simulink model "anim_tp_comde_NL"  (R2016a)
settings: Solver=ode5  SolverMode=SingleTasking  StartTime=0  StopTime=12  FixedStep=.005  MaxStep=0.02  RelTol=1e-3  AbsTol=1e-6
values from neighbouring files (symbols this model uses):
  F = acker(A,B,P)    [Model.m]
  K2 = -256/31.36    (= -8.16326530612)    [Model.m]
  L = 1    [Model.m]
  m = 0.5    [Model.m]
  M = 5    [Model.m]
undefined symbols (not defined in the file): g, X0
settings Model: Creator=user  LastModifiedBy=NADOUR
settings DataIOCC: ExternalInput=[]  InitialState=[]  SaveFormat=Array  SignalLoggingSaveFormat=ModelDataLogs  SaveOutput=off  SaveTime=off
settings OptimizationCC: BooleanDataType=off  ExpressionDepthLimit=2147483647  InitFltsAndDblsToZero=on
settings DebuggingCC: SaveWithParameterizedLinksMsg=none  UnderspecifiedInitializationDetection=Classic  MergeDetectMultiDrivingBlocksExec=none  SignalResolutionControl=TryResolveAllWithWarning  MultiTaskDSMMsg=warning  MultiTaskCondExecSysMsg=none  FcnCallInpInsideContextMsg=UseLocalSettings  StateNameClashWarn=warning
settings HardwareCC: ProdBitPerPointer=32  ProdLargestAtomicFloat=None  ProdIntDivRoundTo=Undefined  ProdEndianess=Unspecified  ProdWordSize=32  ProdHWDeviceType=32-bit Generic  TargetUnknown=on
settings ModelReferenceCC: PropagateSignalLabelsOutOfModel=off
settings GRTTargetCC: TargetFcnLib=ansi_tfl_tmw.mat  CombineOutputUpdateFcns=off  GRTInterface=on
settings ConfigComp: CovModelRefEnable=Off

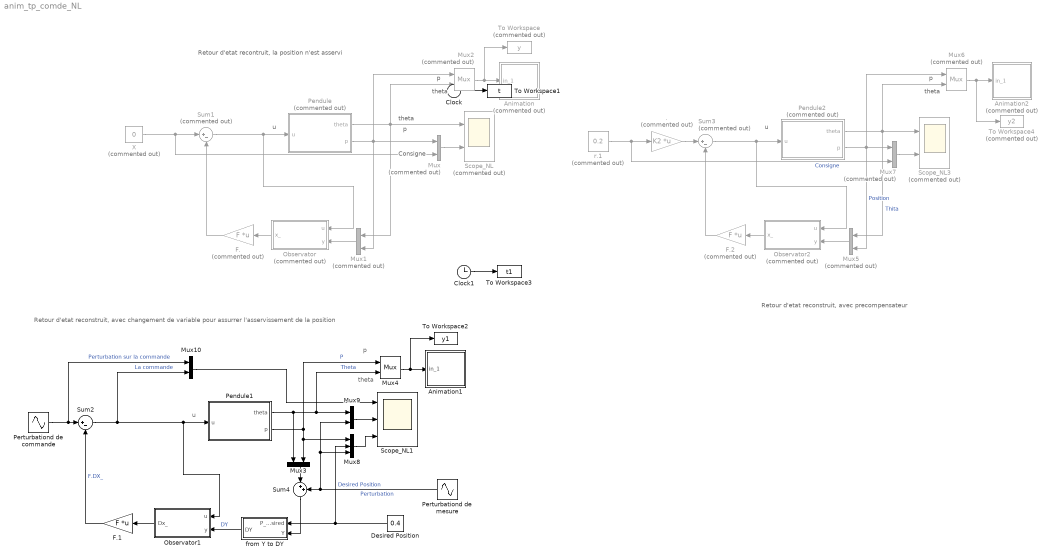
== system anim_tp_comde_NL ==
  note: Retour d'etat reconstruit, avec precompensateur
  note: Retour d'etat reconstruit, avec changement de variable pour assurrer l'asservissement de la position
  note: Retour d'etat recontruit, la position n'est asservi
  note: theta
  note: p
  note: theta
  note: p
  note: u
  note: Consigne
  note: theta
  note: p
  note: u
  note: theta
  note: p
  note: u
  . : Gain  Commented=on  Gain=K2  Multiplication=Matrix(K*u) (u vector)
  Animation : Subsystem  Commented=on  mask(Animation du déplacement du pendule inverse){}
      mask Help: Fonction d'animation du pendule inverse (voir s_fonction tp_pendan_g.m.
      mask Display: plot([-10 10],[0 0],[-2 -2 2 2],[0 1 1 0],[0 -3],[1 5])
  Animation1 : Subsystem  mask(Animation du déplacement du pendule inverse){}
      mask Help: Fonction d'animation du pendule inverse (voir s_fonction tp_pendan_g.m.
      mask Display: plot([-10 10],[0 0],[-2 -2 2 2],[0 1 1 0],[0 -3],[1 5])
  Animation2 : Subsystem  Commented=on  mask(Animation du déplacement du pendule inverse){}
      mask Help: Fonction d'animation du pendule inverse (voir s_fonction tp_pendan_g.m.
      mask Display: plot([-10 10],[0 0],[-2 -2 2 2],[0 1 1 0],[0 -3],[1 5])
  Clock : Clock
  Clock1 : Clock
  Desired Position : Constant  Value=0.4
  F. : Gain  Commented=on  Gain=F  Multiplication=Matrix(K*u) (u vector)
  F.1 : Gain  Gain=F  Multiplication=Matrix(K*u) (u vector)
  F.2 : Gain  Commented=on  Gain=F  Multiplication=Matrix(K*u) (u vector)
  Mux{,1..2,5..7} (6 alike) : Mux  Commented=on  Inputs=2
  Mux{3..4,9..10} (4 alike) : Mux  Inputs=2
  Mux8 : Mux  Inputs=3
  Observator : Subsystem  Commented=on
  Observator1 : Subsystem
  Observator2 : Subsystem  Commented=on
  Pendule : Subsystem  Commented=on  mask(Pendule inverse sur un chariot (éq. Non Linéaires)){M=M, m=m, l=L, g=g, x0=X0}
      mask prompts: M "Masse du chariot (kg):"; m "Masse du pendule (kg):"; l "Longueur de la barre (m):"; g "gravité (m/s^2):"; x0 "Conditions Initiales [theta theta' p p']"
      mask help: Utiliser le menu "Look under mask" pour voir les équations de la dynamique (celles de l'énoncé du TP)
      mask Help: Description Non Linéaire de la dynamique d'un pendule inverse sur un chariot.
      mask Display:
      | plot([-10 10],[1 1],[-2 -2 2 2],[1 2 2 1],[0 3],[2 5])
      | text(-13,0.5,'Eq. Non Linéaires')
      | plot([-14 14],[-0.5 -0.5])
  Pendule1 : Subsystem  mask(Pendule inverse sur un chariot (éq. Non Linéaires)){M=M, m=m, l=L, g=g, x0=X0}
      mask prompts: M "Masse du chariot (kg):"; m "Masse du pendule (kg):"; l "Longueur de la barre (m):"; g "gravité (m/s^2):"; x0 "Conditions Initiales [theta theta' p p']"
      mask help: Utiliser le menu "Look under mask" pour voir les équations de la dynamique (celles de l'énoncé du TP)
      mask Help: Description Non Linéaire de la dynamique d'un pendule inverse sur un chariot.
      mask Display:
      | plot([-10 10],[1 1],[-2 -2 2 2],[1 2 2 1],[0 3],[2 5])
      | text(-13,0.5,'Eq. Non Linéaires')
      | plot([-14 14],[-0.5 -0.5])
  Pendule2 : Subsystem  Commented=on  mask(Pendule inverse sur un chariot (éq. Non Linéaires)){M=M, m=m, l=L, g=g, x0=X0}
      mask prompts: M "Masse du chariot (kg):"; m "Masse du pendule (kg):"; l "Longueur de la barre (m):"; g "gravité (m/s^2):"; x0 "Conditions Initiales [theta theta' p p']"
      mask help: Utiliser le menu "Look under mask" pour voir les équations de la dynamique (celles de l'énoncé du TP)
      mask Help: Description Non Linéaire de la dynamique d'un pendule inverse sur un chariot.
      mask Display:
      | plot([-10 10],[1 1],[-2 -2 2 2],[1 2 2 1],[0 3],[2 5])
      | text(-13,0.5,'Eq. Non Linéaires')
      | plot([-14 14],[-0.5 -0.5])
  Perturbationd de commande : Sin  Amplitude=0.1  Frequency=0.1  SampleTime=0
  Perturbationd de mesure : Sin  Amplitude=0.2  Frequency=100  SampleTime=0
  Scope_NL : Scope  Commented=on  NumInputPorts=2
  Scope_NL1 : Scope  NumInputPorts=3
  Scope_NL3 : Scope  Commented=on  NumInputPorts=2
  Sum1 : Sum  Commented=on  Inputs=|+-
  Sum2 : Sum  Inputs=|+-
  Sum3 : Sum  Commented=on  Inputs=|+-
  Sum4 : Sum  Inputs=|++
  To Workspace : ToWorkspace  Commented=on  VariableName=y  SampleTime=0.1
  To Workspace1 : ToWorkspace  VariableName=t  SampleTime=0.1
  To Workspace2 : ToWorkspace  VariableName=y1  SampleTime=0.1
  To Workspace3 : ToWorkspace  VariableName=t1  SampleTime=0.1
  To Workspace4 : ToWorkspace  Commented=on  VariableName=y2  SampleTime=0.1
  X : Constant  Commented=on  Value=0
  from Y to DY : MATLAB Function  TreatAsAtomicUnit=on
  r.1 : Constant  Commented=on  Value=0.2
  wires:
  Mux2/1 -> To Workspace/1, Animation/1(in_1)
  Clock/1 -> To Workspace1/1
  Pendule/2(p) -> Mux/1, Mux1/2, Mux2/1
  Pendule/1(theta) -> Mux1/1, Mux2/2, Scope_NL/1
  Observator/1(x_) -> F./1
  Mux1/1 -> Observator/2(y)
  Sum1/1 -> Observator/1(u), Pendule/1(u)
  F./1 -> Sum1/2
  X/1 -> Mux/2, Sum1/1
  Mux4/1 -> To Workspace2/1, Animation1/1(in_1)
  Clock1/1 -> To Workspace3/1
  Pendule1/2(p) -> Mux8/1, Mux3/2, Mux4/1  "P"
  Pendule1/1(theta) -> Mux4/2, Mux9/1, Mux3/1  "Theta"
  Observator1/1(Dx_) -> F.1/1
  Sum4/1 -> from Y to DY/2(Y)
  Sum2/1 -> Mux10/2, Observator1/1(u), Pendule1/1(u)  "La commande"
  F.1/1 -> Sum2/2  "F.DX_"
  from Y to DY/1(DY) -> Observator1/2(y)  "DY"
  Desired Position/1 -> from Y to DY/1(P_desired), Mux8/2  "Desired Position"
  Mux6/1 -> Animation2/1(in_1), To Workspace4/1
  Pendule2/2(p) -> Mux5/2, Mux7/1, Mux6/1  "Position"
  Pendule2/1(theta) -> Mux5/1, Scope_NL3/1, Mux6/2  "Thita"
  Observator2/1(x_) -> F.2/1
  Mux5/1 -> Observator2/2(y)
  Sum3/1 -> Pendule2/1(u), Observator2/1(u)
  F.2/1 -> Sum3/2
  ./1 -> Sum3/1
  r.1/1 -> Mux7/2, ./1  "Consigne"
  Mux/1 -> Scope_NL/2
  Mux7/1 -> Scope_NL3/2
  Mux3/1 -> Sum4/1
  Perturbationd de mesure/1 -> Mux9/2, Mux8/3, Sum4/2  "Perturbation"
  Perturbationd de commande/1 -> Mux10/1, Sum2/1  "Perturbation sur la commande"
  Mux9/1 -> Scope_NL1/2
  Mux8/1 -> Scope_NL1/3
  Mux10/1 -> Scope_NL1/1

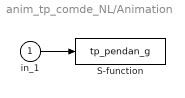
== system anim_tp_comde_NL/Animation ==
  in_1 : Inport
  S-function : S-Function  FunctionName=tp_pendan_g  SFunctionDeploymentMode=off  EnableBusSupport=off
      settings: DeleteFcn=pendan([],[],[],'DeleteBlock');
  wires:
  in_1/1 -> S-function/1

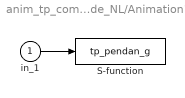
== system anim_tp_comde_NL/Animation1 ==
  in_1 : Inport
  S-function : S-Function  FunctionName=tp_pendan_g  SFunctionDeploymentMode=off  EnableBusSupport=off
      settings: DeleteFcn=pendan([],[],[],'DeleteBlock');
  wires:
  in_1/1 -> S-function/1

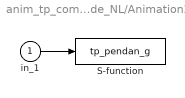
== system anim_tp_comde_NL/Animation2 ==
  in_1 : Inport
  S-function : S-Function  FunctionName=tp_pendan_g  SFunctionDeploymentMode=off  EnableBusSupport=off
      settings: DeleteFcn=pendan([],[],[],'DeleteBlock');
  wires:
  in_1/1 -> S-function/1

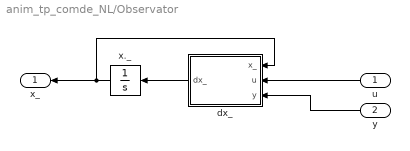
== system anim_tp_comde_NL/Observator ==
  u : Inport
  y : Inport  Port=2
  dx_ : MATLAB Function  TreatAsAtomicUnit=on
  x._ : Integrator
  x_ : Outport
  wires:
  u/1 -> dx_/2(u)
  y/1 -> dx_/3(y)
  dx_/1(dx_) -> x._/1
  x._/1 -> x_/1, dx_/1(x_)

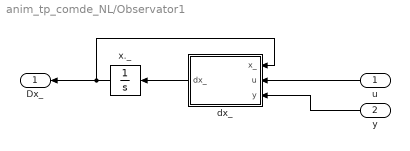
== system anim_tp_comde_NL/Observator1 ==
  u : Inport
  y : Inport  Port=2
  dx_ : MATLAB Function  TreatAsAtomicUnit=on
  x._ : Integrator
  Dx_ : Outport
  wires:
  u/1 -> dx_/2(u)
  y/1 -> dx_/3(y)
  dx_/1(dx_) -> x._/1
  x._/1 -> Dx_/1, dx_/1(x_)

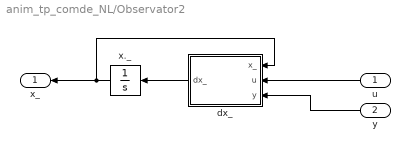
== system anim_tp_comde_NL/Observator2 ==
  u : Inport
  y : Inport  Port=2
  dx_ : MATLAB Function  TreatAsAtomicUnit=on
  x._ : Integrator
  x_ : Outport
  wires:
  x._/1 -> dx_/1(x_), x_/1
  dx_/1(dx_) -> x._/1
  y/1 -> dx_/3(y)
  u/1 -> dx_/2(u)

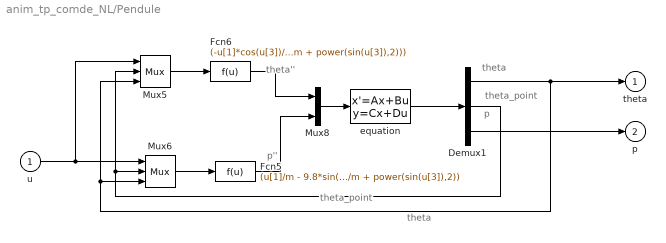
== system anim_tp_comde_NL/Pendule ==
  note: theta
  note: theta_point
  note: p''
  note: theta''
  note: theta
  note: theta_point
  note: p
  u : Inport
  Demux1 : Demux  Outputs=3
  Fcn5 : Fcn  Expr=(u[1]/m - 9.8*sin(u[3])*cos(u[3]) + L*power(u[2],2)*sin(u[3]))/(M/m + power(sin(u[3]),2))
  Fcn6 : Fcn  Expr=(-u[1]*cos(u[3])/m + (M+m)*9.8*sin(u[3])/m - L*power(u[2],2)*sin(u[3])*cos(u[3]))/(l*(M/m + power(sin(u[3]),2)))
  Mux5 : Mux  Inputs=3
  Mux6 : Mux  Inputs=3
  Mux8 : Mux  Inputs=2
  equation : StateSpace  A=[ 0 1 0 0 ; 0 0 0 0 ; 0 0 0 1; 0 0 0 0]  B=[0 0 ; 1 0 ; 0 0 ; 0 1]  C=[1 0 0 0 ; 0 1 0 0 ; 0 0 1 0]  D=zeros(3,2)  X0=x0
  theta : Outport  InitialOutput=0
  p : Outport  Port=2  InitialOutput=0
  wires:
  u/1 -> Mux6/1, Mux5/1
  Mux6/1 -> Fcn5/1
  Mux5/1 -> Fcn6/1
  Demux1/2 -> Mux5/2, Mux6/2
  equation/1 -> Demux1/1
  Fcn6/1 -> Mux8/1
  Fcn5/1 -> Mux8/2
  Mux8/1 -> equation/1
  Demux1/1 -> Mux6/3, Mux5/3, theta/1
  Demux1/3 -> p/1

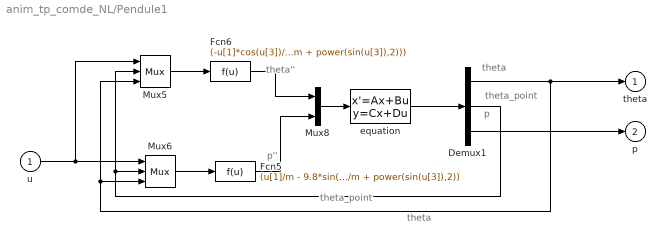
== system anim_tp_comde_NL/Pendule1 ==
  note: theta
  note: theta_point
  note: p''
  note: theta''
  note: theta
  note: theta_point
  note: p
  u : Inport
  Demux1 : Demux  Outputs=3
  Fcn5 : Fcn  Expr=(u[1]/m - 9.8*sin(u[3])*cos(u[3]) + L*power(u[2],2)*sin(u[3]))/(M/m + power(sin(u[3]),2))
  Fcn6 : Fcn  Expr=(-u[1]*cos(u[3])/m + (M+m)*9.8*sin(u[3])/m - L*power(u[2],2)*sin(u[3])*cos(u[3]))/(l*(M/m + power(sin(u[3]),2)))
  Mux5 : Mux  Inputs=3
  Mux6 : Mux  Inputs=3
  Mux8 : Mux  Inputs=2
  equation : StateSpace  A=[ 0 1 0 0 ; 0 0 0 0 ; 0 0 0 1; 0 0 0 0]  B=[0 0 ; 1 0 ; 0 0 ; 0 1]  C=[1 0 0 0 ; 0 1 0 0 ; 0 0 1 0]  D=zeros(3,2)  X0=x0
  theta : Outport  InitialOutput=0
  p : Outport  Port=2  InitialOutput=0
  wires:
  u/1 -> Mux6/1, Mux5/1
  Mux6/1 -> Fcn5/1
  Mux5/1 -> Fcn6/1
  Demux1/2 -> Mux5/2, Mux6/2
  equation/1 -> Demux1/1
  Fcn6/1 -> Mux8/1
  Fcn5/1 -> Mux8/2
  Mux8/1 -> equation/1
  Demux1/1 -> Mux6/3, Mux5/3, theta/1
  Demux1/3 -> p/1

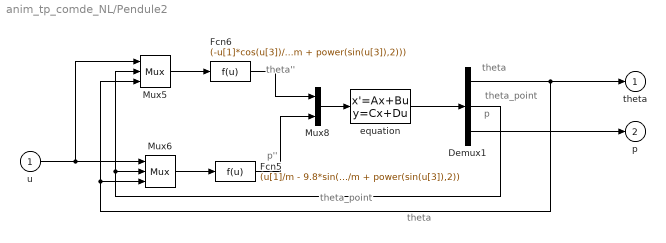
== system anim_tp_comde_NL/Pendule2 ==
  note: p
  note: theta_point
  note: theta
  note: theta''
  note: p''
  note: theta_point
  note: theta
  u : Inport
  Demux1 : Demux  Outputs=3
  Fcn5 : Fcn  Expr=(u[1]/m - 9.8*sin(u[3])*cos(u[3]) + L*power(u[2],2)*sin(u[3]))/(M/m + power(sin(u[3]),2))
  Fcn6 : Fcn  Expr=(-u[1]*cos(u[3])/m + (M+m)*9.8*sin(u[3])/m - L*power(u[2],2)*sin(u[3])*cos(u[3]))/(l*(M/m + power(sin(u[3]),2)))
  Mux5 : Mux  Inputs=3
  Mux6 : Mux  Inputs=3
  Mux8 : Mux  Inputs=2
  equation : StateSpace  A=[ 0 1 0 0 ; 0 0 0 0 ; 0 0 0 1; 0 0 0 0]  B=[0 0 ; 1 0 ; 0 0 ; 0 1]  C=[1 0 0 0 ; 0 1 0 0 ; 0 0 1 0]  D=zeros(3,2)  X0=x0
  theta : Outport  InitialOutput=0
  p : Outport  Port=2  InitialOutput=0
  wires:
  Demux1/3 -> p/1
  Demux1/1 -> theta/1, Mux5/3, Mux6/3
  Mux8/1 -> equation/1
  Fcn5/1 -> Mux8/2
  Fcn6/1 -> Mux8/1
  equation/1 -> Demux1/1
  Demux1/2 -> Mux6/2, Mux5/2
  Mux5/1 -> Fcn6/1
  Mux6/1 -> Fcn5/1
  u/1 -> Mux5/1, Mux6/1

== matlab function anim_tp_comde_NL/Observator1/dx_ ==
  data: x_ input; u input; y input; dx_ output
function dx_=f(x_,u,y)
%% Parameteres:
m=0.5; M=5; L=1; g=9.8;

%% 1) The Model:
A = [0          1 0 0
    g*(m+M)/M/L 0 0 0
    0           0 0 1
    -m*g/M      0 0 0];

B = [0 ; -1/M/L; 0; 1/M];

C= [1 0 0 0
    0 0 1 0];
K =[2.9998   -0.9985
   14.7801    0.0043
    1.0015    3.0002
   -0.9757    3.9999];
%% The observation
y_=C*x_;
dx_= A*x_ + B*u + K*(y-y_);

== matlab function anim_tp_comde_NL/Observator/dx_ ==
  data: x_ input; u input; y input; dx_ output
function dx_=f(x_,u,y)
%% Parameteres:
m=0.5; M=5; L=1; g=9.8;

%% 1) The Model:
A = [0          1 0 0
    g*(m+M)/M/L 0 0 0
    0           0 0 1
    -m*g/M      0 0 0];

B = [0 ; -1/M/L; 0; 1/M];

C= [1 0 0 0
    0 0 1 0];
K =[2.9998   -0.9985
   14.7801    0.0043
    1.0015    3.0002
   -0.9757    3.9999];
%% The observation
y_=C*x_;
dx_= A*x_ + B*u + K*(y-y_);

== matlab function anim_tp_comde_NL/from Y to DY ==
  data: P_desired input; DY output; Y input
function DY = fct(P_desired,Y)

DY = Y-[0; P_desired];

== matlab function anim_tp_comde_NL/Observator2/dx_ ==
  data: x_ input; u input; y input; dx_ output
function dx_=f(x_,u,y)
%% Parameteres:
m=0.5; M=5; L=1; g=9.8;

%% 1) The Model:
A = [0          1 0 0
    g*(m+M)/M/L 0 0 0
    0           0 0 1
    -m*g/M      0 0 0];

B = [0 ; -1/M/L; 0; 1/M];

C= [1 0 0 0
    0 0 1 0];
K =[2.9998   -0.9985
   14.7801    0.0043
    1.0015    3.0002
   -0.9757    3.9999];
%% The observation
y_=C*x_;
dx_= A*x_ + B*u + K*(y-y_);
